simulink model "gradient_estimator"  (R2024b)
settings: Solver=VariableStepAuto  StartTime=0.0  StopTime=50  MaxStep=1E-1  RelTol=1e-3
model workspace (MAT data in the model file):
  g = -5
settings Model: Creator=djd14  LastModifiedBy=djd14

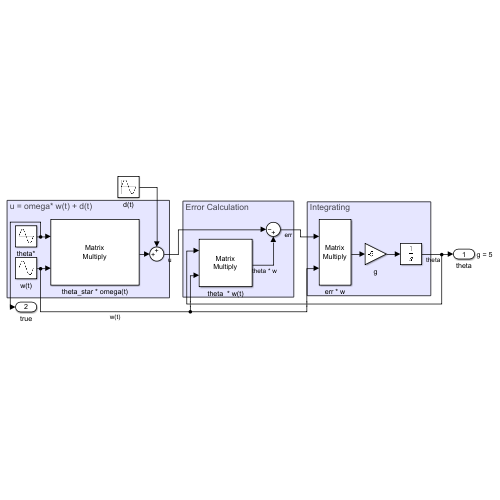
[thumbnail: Simulink's stored preview of the top-level diagram]
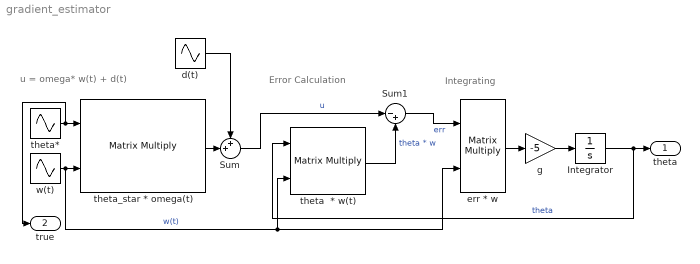
== system gradient_estimator ==
  note: Integrating
  note: Error Calculation
  note: u = omega* w(t) + d(t)
  Integrator : Integrator
  Sum : Sum  Inputs=++|
  Sum1 : Sum  Inputs=|-+
  d(t) : Sin  Amplitude=0  Frequency=20  SampleTime=0
  err * w : Product  Multiplication=Matrix(*)
  g : Gain  Gain=-5
  theta  * w(t) : Product  Multiplication=Matrix(*)
  theta* : Sin  Amplitude=0.5  Bias=1  Frequency=0.5  SampleTime=0
  theta_star * omega(t) : Product  Multiplication=Matrix(*)
  w(t) : Sin  SampleTime=0
  theta : Outport  SignalName=g = 5
  true : Outport  Port=2
  wires:
  Sum/1 -> Sum1/1  "u"
  theta_star * omega(t)/1 -> Sum/2
  theta*/1 -> true/1, theta_star * omega(t)/1
  d(t)/1 -> Sum/1
  w(t)/1 -> err * w/2, theta  * w(t)/2, theta_star * omega(t)/2  "w(t)"
  Sum1/1 -> err * w/1  "err"
  theta  * w(t)/1 -> Sum1/2  "theta * w"
  Integrator/1 -> theta/1, theta  * w(t)/1  "theta"
  g/1 -> Integrator/1
  err * w/1 -> g/1
